simulink library "UAVdesign_net"  (Simulink 7.7)
settings: Solver=ode45  SolverMode=SingleTasking  StartTime=0.0  StopTime=10.0  RelTol=1e-3
undefined symbols (not defined in the file or in its folder): alpha_IERA_IELA_IELA, R_IERA_RA_RA
libraries: UAVdesign_net x75, simulink x13
(part 2 of 8)

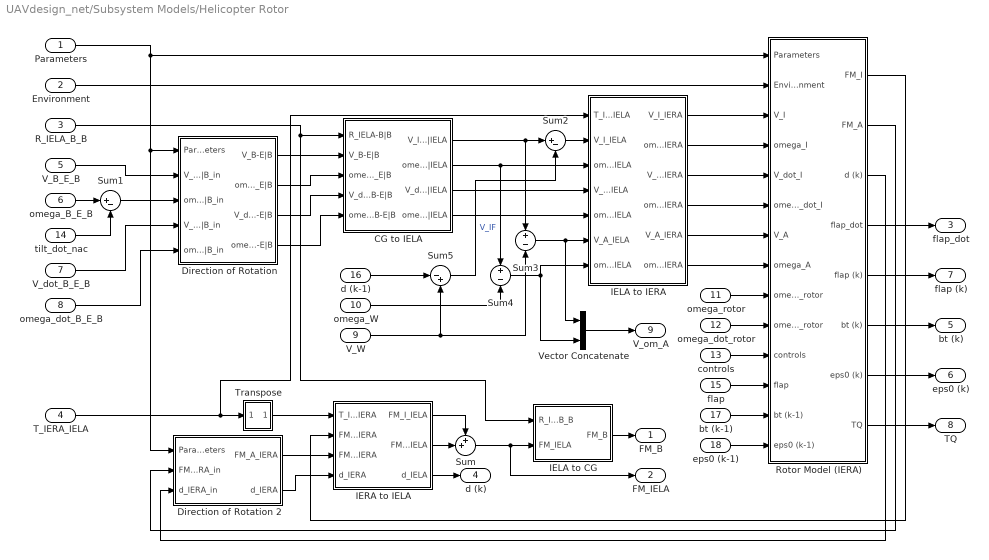
== system UAVdesign_net/Subsystem Models/Helicopter Rotor ==
  Parameters : Inport  OutDataTypeStr=Bus: RotorParameters
  Environment : Inport  Port=2  OutDataTypeStr=Bus: Environment
  R_IELA_B_B : Inport  Port=3  PortDimensions=3
  T_IERA_IELA : Inport  Port=4  PortDimensions=[3 3]
  V_B_E_B : Inport  Port=5  PortDimensions=3
  omega_B_E_B : Inport  Port=6  PortDimensions=3
  V_dot_B_E_B : Inport  Port=7  PortDimensions=3
  omega_dot_B_E_B : Inport  Port=8  PortDimensions=3
  V_W : Inport  Port=9  PortDimensions=3
  omega_W : Inport  Port=10  PortDimensions=3
  omega_rotor : Inport  Port=11  PortDimensions=1
  omega_dot_rotor : Inport  Port=12  PortDimensions=1
  controls : Inport  Port=13  PortDimensions=3
  tilt_dot_nac : Inport  Port=14  PortDimensions=3
  flap : Inport  Port=15  PortDimensions=3
  d (k-1) : Inport  Port=16  PortDimensions=3
  bt (k-1) : Inport  Port=17  PortDimensions=1
  eps0 (k-1) : Inport  Port=18  PortDimensions=1
  CG to IELA : Subsystem
      mask Display:
      | port_label('input', 1, 'R_{IELA-B|B}', 'texmode', 'on')
      | port_label('input', 2, 'V_{B-E|B}', 'texmode', 'on')
      | port_label('input', 3, '\omega_{B-E|B}', 'texmode', 'on')
      | port_label('input', 4, 'V^\bullet_{B-E|B}', 'texmode', 'on')
      | port_label('input', 5, '\omega^\bullet_{B-E|B}', 'texmode', 'on')
      | port_label('output', 1, 'V_{IELA-E|IELA}', 'texmode', 'on')
      | port_label('output', 2, '\omega_{IELA-E|IELA}', 'texmode', 'on')
      | port_label('output', 3, 'V^\bullet_{IELA-E|IELA}', 'texmode', 'on')
      | port_label('output', 4, '\omega^\bullet_{IELA-E|IELA}', 'texmode', 'on')
  Direction of Rotation : Subsystem
      mask Display:
      | port_label('input', 1, 'Parameters', 'texmode', 'on')
      | port_label('input', 2, 'V_{B-E|B}', 'texmode', 'on')
      | port_label('input', 3, '\omega_{B-E|B}', 'texmode', 'on')
      | port_label('input', 4, 'V^\bullet_{B-E|B}', 'texmode', 'on')
      | port_label('input', 5, '\omega^\bullet_{B-E|B}', 'texmode', 'on')
      | port_label('output', 1, 'V_{B-E|B}', 'texmode', 'on')
      | port_label('output', 2, '\omega_{B-E|B}', 'texmode', 'on')
      | port_label('output', 3, 'V^\bullet_{B-E|B}', 'texmode', 'on')
      | port_label('output', 4, '\omega^\bullet_{B-E|B}', 'texmode', 'on')
  Direction of Rotation 2 : Subsystem
      mask Display:
      | port_label('input', 1, 'Parameters', 'texmode', 'on')
      | port_label('input', 2, 'FM_{A|IERA}', 'texmode', 'on')
      | port_label('input', 3, 'd_{IERA}', 'texmode', 'on')
      | port_label('output', 1, 'FM_{A|IERA}', 'texmode', 'on')
      | port_label('output', 2, 'd_{IERA}', 'texmode', 'on')
  IELA to CG : Subsystem
      mask Display:
      | port_label('input', 1, 'R_{IELA-B|B}', 'texmode', 'on')
      | port_label('input', 2, 'FM_{IELA}', 'texmode', 'on')
      | port_label('output', 1, 'FM_{B}', 'texmode', 'on')
  IELA to IERA : Subsystem
      mask Display:
      | port_label('input', 1, 'T_{IERA-IELA}', 'texmode', 'on')
      | port_label('input', 2, 'V_{I|IELA}', 'texmode', 'on')
      | port_label('input', 3, '\omega_{I|IELA}', 'texmode', 'on')
      | port_label('input', 4, 'V^\bullet_{I|IELA}', 'texmode', 'on')
      | port_label('input', 5, '\omega^\bullet_{I|IELA}', 'texmode', 'on')
      | port_label('input', 6, 'V_{A|IELA}', 'texmode', 'on')
      | port_label('input', 7, '\omega_{A|IELA}', 'texmode', 'on')
      | 
      | port_label('output', 1, 'V_{I|IERA}', 'texmode', 'on')
      | port_label('output', 2, '\omega_{I|IERA}', 'texmode', 'on')
      | port_label('output', 3, 'V^\bullet_{I|IERA}', 'texmode', 'on')
      | port_label('output', 4, '\omega^\bullet_{I|IERA}', 'texmode', 'on')
      | port_label('output', 5, 'V_{A|IERA}', 'texmode', 'on')
      | port_label('output', 6, '\omega_{A|IERA}', 'texmode', 'on')
  IERA to IELA : Subsystem
      mask Display:
      | port_label('input', 1, 'T_{IELA-IERA}', 'texmode', 'on')
      | port_label('input', 2, 'FM_{I|IERA}', 'texmode', 'on')
      | port_label('input', 3, 'FM_{A|IERA}', 'texmode', 'on')
      | port_label('input', 4, 'd_{IERA}', 'texmode', 'on')
      | port_label('output', 1, 'FM_{I|IELA}', 'texmode', 'on')
      | port_label('output', 2, 'FM_{A|IELA}', 'texmode', 'on')
      | port_label('output', 3, 'd_{IELA}', 'texmode', 'on')
  Rotor Model (IERA) : Subsystem
      mask Display:
      | port_label('input', 1, 'Parameters', 'texmode', 'on')
      | port_label('input', 2, 'Environment', 'texmode', 'on')
      | port_label('input', 3, 'V_{I}', 'texmode', 'on')
      | port_label('input', 4, '\omega_{I}', 'texmode', 'on')
      | port_label('input', 5, 'V^\bullet_{I}', 'texmode', 'on')
      | port_label('input', 6, '\omega^\bullet_{I}', 'texmode', 'on')
      | port_label('input', 7, 'V_{A}', 'texmode', 'on')
      | port_label('input', 8, '\omega_{A}', 'texmode', 'on')
      | port_label('input', 9, '\Omega_{rotor}', 'texmode', 'on')
      | port_label('input', 10, '\Omega^\bullet_{rotor}', 'texmode', 'on')
      | port_label('input', 11, 'controls', 'texmode', 'on')
      | port_label('input', 12, 'flap', 'texmode', 'on')
      | port_label('input', 13, 'bt_{k-1}', 'texmode', 'on')
      | port_label('input', 14, 'eps0_{k-1}', 'texmode', 'on')
      | 
      | port_label('output', 1, 'FM_{I}', 'texmode', 'on')
      | port_label('output', 2, 'FM_{A}', 'texmode', 'on')
      | port_label('output', 3, 'd_{k}', 'texmode', 'on')
      | port_label('output', 4, 'flap^\bullet', 'texmode', 'on')
      | port_label('output', 5, 'flap_{k}', 'texmode', 'on')
      | port_label('output', 6, 'bt_{k}', 'texmode', 'on')
      | port_label('output', 7, 'eps0_{k}', 'texmode', 'on')
      | port_label('output', 8, 'Lift & Torque', 'texmode', 'on')
  Sum : Sum  Inputs=++|
  Sum1 : Sum  Inputs=|+-
  Sum2 : Sum  Inputs=|+-
  Sum3 : Sum  Inputs=+|-
  Sum4 : Sum  Inputs=+|-
  Sum5 : Sum  Inputs=|-+
  Transpose : Subsystem
      mask Display: disp('A^T', 'texmode', 'on')
  Vector Concatenate : Concatenate  Mode=Vector
  FM_B : Outport  PortDimensions=6
  FM_IELA : Outport  Port=2  PortDimensions=6
  flap_dot : Outport  Port=3  PortDimensions=3
  d (k) : Outport  Port=4  PortDimensions=3
  bt (k) : Outport  Port=5  PortDimensions=1
  eps0 (k) : Outport  Port=6  PortDimensions=1
  flap (k) : Outport  Port=7  PortDimensions=3
  TQ : Outport  Port=8  PortDimensions=2
  V_om_A : Outport  Port=9  PortDimensions=6
  wires:
  R_IELA_B_B/1 -> CG to IELA/1(R_IELA-B|B), IELA to CG/1(R_IELA_B_B)
  eps0 (k-1)/1 -> Rotor Model (IERA)/14(eps0 (k-1))
  IERA to IELA/3(d_IELA) -> d (k)/1
  Rotor Model (IERA)/7(eps0 (k)) -> eps0 (k)/1
  bt (k-1)/1 -> Rotor Model (IERA)/13(bt (k-1))
  IELA to CG/1(FM_B) -> FM_B/1
  Transpose/1(Out) -> IERA to IELA/1(T_IELA_IERA)
  Rotor Model (IERA)/6(bt (k)) -> bt (k)/1
  flap/1 -> Rotor Model (IERA)/12(flap)
  controls/1 -> Rotor Model (IERA)/11(controls)
  Rotor Model (IERA)/5(flap (k)) -> flap (k)/1
  omega_dot_rotor/1 -> Rotor Model (IERA)/10(omega_dot_rotor)
  omega_W/1 -> Sum4/2
  omega_rotor/1 -> Rotor Model (IERA)/9(omega_rotor)
  d (k-1)/1 -> Sum5/1
  Rotor Model (IERA)/4(flap_dot) -> flap_dot/1
  omega_dot_B_E_B/1 -> Direction of Rotation/5(omega_dot_B-E|B_in)
  tilt_dot_nac/1 -> Sum1/2
  V_dot_B_E_B/1 -> Direction of Rotation/4(V_dot_B-E|B_in)
  omega_B_E_B/1 -> Sum1/1
  V_B_E_B/1 -> Direction of Rotation/2(V_B-E|B_in)
  T_IERA_IELA/1 -> Transpose/1(In), IELA to IERA/1(T_IERA_IELA)
  Environment/1 -> Rotor Model (IERA)/2(Environment)
  Parameters/1 -> Direction of Rotation 2/1(Parameters), Direction of Rotation/1(Parameters), Rotor Model (IERA)/1(Parameters)
  Direction of Rotation 2/2(d_IERA) -> IERA to IELA/4(d_IERA)
  Rotor Model (IERA)/3(d (k)) -> Direction of Rotation 2/3(d_IERA_in)
  Sum5/1 -> Sum2/2  "V_IF"
  Direction of Rotation 2/1(FM_A_IERA) -> IERA to IELA/3(FM_A_IERA)
  IERA to IELA/2(FM_A_IELA) -> Sum/2
  IELA to IERA/6(omega_A_IERA) -> Rotor Model (IERA)/8(omega_A)
  IELA to IERA/5(V_A_IERA) -> Rotor Model (IERA)/7(V_A)
  IELA to IERA/4(omega_dot_I_IERA) -> Rotor Model (IERA)/6(omega_dot_I)
  IELA to IERA/3(V_dot_I_IERA) -> Rotor Model (IERA)/5(V_dot_I)
  IELA to IERA/2(omega_I_IERA) -> Rotor Model (IERA)/4(omega_I)
  IELA to IERA/1(V_I_IERA) -> Rotor Model (IERA)/3(V_I)
  Sum4/1 -> IELA to IERA/7(omega_A_IELA), Vector Concatenate/2
  V_W/1 -> Sum5/2, Sum3/2
  Sum3/1 -> IELA to IERA/6(V_A_IELA), Vector Concatenate/1
  Sum2/1 -> IELA to IERA/2(V_I_IELA)
  CG to IELA/1(V_IELA-E|IELA) -> Sum3/1, Sum2/1
  Direction of Rotation/4(omega_dot_B-E|B) -> CG to IELA/5(omega_dot_B-E|B)
  Direction of Rotation/3(V_dot_B-E|B) -> CG to IELA/4(V_dot_B-E|B)
  Direction of Rotation/2(omega_B_E|B) -> CG to IELA/3(omega_B_E|B)
  Direction of Rotation/1(V_B-E|B) -> CG to IELA/2(V_B-E|B)
  Sum1/1 -> Direction of Rotation/3(omega_B_E|B_in)
  Rotor Model (IERA)/1(FM_I) -> IERA to IELA/2(FM_I_IERA)
  Rotor Model (IERA)/2(FM_A) -> Direction of Rotation 2/2(FM_A_IERA_in)
  Sum/1 -> IELA to CG/2(FM_IELA), FM_IELA/1
  IERA to IELA/1(FM_I_IELA) -> Sum/1
  CG to IELA/4(omega_dot_IELA-E|IELA) -> IELA to IERA/5(omega_dot_I_IELA)
  CG to IELA/3(V_dot_IELA-E|IELA) -> IELA to IERA/4(V_dot_I_IELA)
  CG to IELA/2(omega_IELA-E|IELA) -> Sum4/1, IELA to IERA/3(omega_I_IELA)
  Rotor Model (IERA)/8(TQ) -> TQ/1
  Vector Concatenate/1 -> V_om_A/1

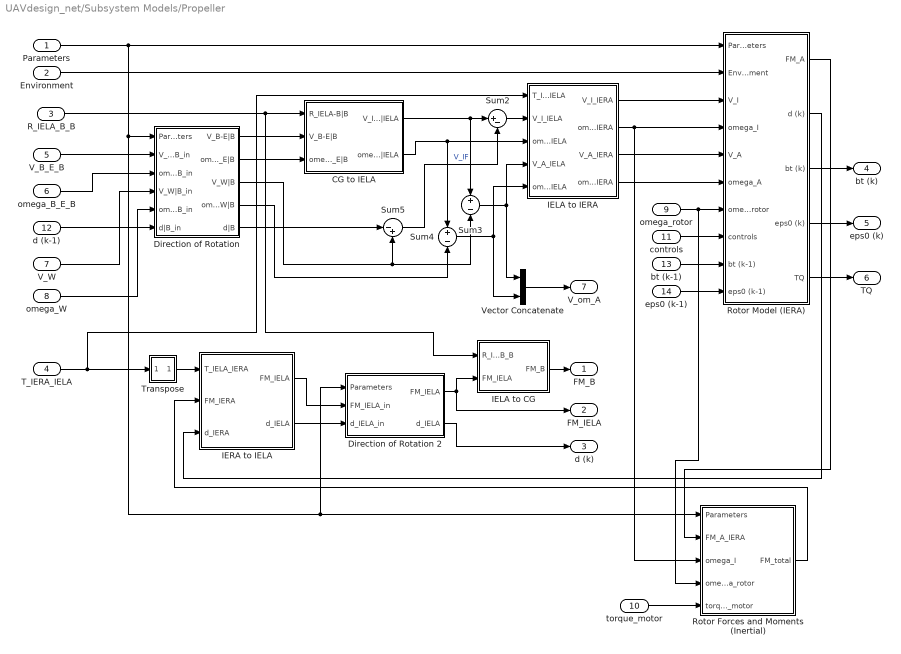
== system UAVdesign_net/Subsystem Models/Propeller ==
  Parameters : Inport
  Environment : Inport  Port=2
  R_IELA_B_B : Inport  Port=3  PortDimensions=3
  T_IERA_IELA : Inport  Port=4  PortDimensions=[3 3]
  V_B_E_B : Inport  Port=5  PortDimensions=3
  omega_B_E_B : Inport  Port=6  PortDimensions=3
  V_W : Inport  Port=7  PortDimensions=3
  omega_W : Inport  Port=8  PortDimensions=3
  omega_rotor : Inport  Port=9  PortDimensions=1
  torque_motor : Inport  Port=10  PortDimensions=1
  controls : Inport  Port=11  PortDimensions=1
  d (k-1) : Inport  Port=12  PortDimensions=3
  bt (k-1) : Inport  Port=13  PortDimensions=1
  eps0 (k-1) : Inport  Port=14  PortDimensions=1
  CG to IELA : Subsystem
      mask Display:
      | port_label('input', 1, 'R_{IELA-B|B}', 'texmode', 'on')
      | port_label('input', 2, 'V_{B-E|B}', 'texmode', 'on')
      | port_label('input', 3, '\omega_{B-E|B}', 'texmode', 'on')
      | port_label('output', 1, 'V_{IELA-E|IELA}', 'texmode', 'on')
      | port_label('output', 2, '\omega_{IELA-E|IELA}', 'texmode', 'on')
  Direction of Rotation : Subsystem
      mask Display:
      | port_label('input', 1, 'Parameters', 'texmode', 'on')
      | port_label('input', 2, 'V_{B-E|B}', 'texmode', 'on')
      | port_label('input', 3, '\omega_{B-E|B}', 'texmode', 'on')
      | port_label('input', 4, 'V_{W|B}', 'texmode', 'on')
      | port_label('input', 5, '\omega_{W|B}', 'texmode', 'on')
      | port_label('input', 6, 'd', 'texmode', 'on')
      | 
      | port_label('output', 1, 'V_{B-E|B}', 'texmode', 'on')
      | port_label('output', 2, '\omega_{B-E|B}', 'texmode', 'on')
      | port_label('output', 3, 'V_{W|B}', 'texmode', 'on')
      | port_label('output', 4, '\omega_{W|B}', 'texmode', 'on')
      | port_label('output', 5, 'd', 'texmode', 'on')
  Direction of Rotation 2 : Subsystem
      mask Display:
      | port_label('input', 1, 'Parameters', 'texmode', 'on')
      | port_label('input', 2, 'FM_{IELA}', 'texmode', 'on')
      | port_label('input', 3, 'd_{IELA}', 'texmode', 'on')
      | port_label('output', 1, 'FM_{IELA}', 'texmode', 'on')
      | port_label('output', 2, 'd_{IELA}', 'texmode', 'on')
  IELA to CG : Subsystem
      mask Display:
      | port_label('input', 1, 'R_{IELA-B|B}', 'texmode', 'on')
      | port_label('input', 2, 'FM_{IELA}', 'texmode', 'on')
      | port_label('output', 1, 'FM_{B}', 'texmode', 'on')
  IELA to IERA : Subsystem
      mask Display:
      | port_label('input', 1, 'T_{IERA-IELA}', 'texmode', 'on')
      | port_label('input', 2, 'V_{I|IELA}', 'texmode', 'on')
      | port_label('input', 3, '\omega_{I|IELA}', 'texmode', 'on')
      | port_label('input', 4, 'V_{A|IELA}', 'texmode', 'on')
      | port_label('input', 5, '\omega_{A|IELA}', 'texmode', 'on')
      | 
      | port_label('output', 1, 'V_{I|IERA}', 'texmode', 'on')
      | port_label('output', 2, '\omega_{I|IERA}', 'texmode', 'on')
      | port_label('output', 3, 'V_{A|IERA}', 'texmode', 'on')
      | port_label('output', 4, '\omega_{A|IERA}', 'texmode', 'on')
  IERA to IELA : Subsystem
      mask Display:
      | port_label('input', 1, 'T_{IELA-IERA}', 'texmode', 'on')
      | port_label('input', 2, 'FM_{IERA}', 'texmode', 'on')
      | port_label('input', 3, 'd_{IERA}', 'texmode', 'on')
      | port_label('output', 1, 'FM_{IELA}', 'texmode', 'on')
      | port_label('output', 2, 'd_{IELA}', 'texmode', 'on')
  Rotor Forces and Moments (Inertial) : Subsystem
      mask Display:
      | port_label('input', 1, 'Parameters', 'texmode', 'on')
      | port_label('input', 2, 'FM_{A|IERA}', 'texmode', 'on')
      | port_label('input', 3, '\omega_{I|IERA}', 'texmode', 'on')
      | port_label('input', 4, '\Omega_{rotor}', 'texmode', 'on')
      | port_label('input', 5, '\tau_{motor}', 'texmode', 'on')
      | 
      | port_label('output', 1, 'FM_{total|IERA}', 'texmode', 'on')
  Rotor Model (IERA) : Subsystem
      mask Display:
      | port_label('input', 1, 'Parameters', 'texmode', 'on')
      | port_label('input', 2, 'Environment', 'texmode', 'on')
      | port_label('input', 3, 'V_{I}', 'texmode', 'on')
      | port_label('input', 4, '\omega_{I}', 'texmode', 'on')
      | port_label('input', 5, 'V_{A}', 'texmode', 'on')
      | port_label('input', 6, '\omega_{A}', 'texmode', 'on')
      | port_label('input', 7, '\Omega_{rotor}', 'texmode', 'on')
      | port_label('input', 8, 'controls', 'texmode', 'on')
      | port_label('input', 9, 'bt_{k-1}', 'texmode', 'on')
      | port_label('input', 10, 'eps0_{k-1}', 'texmode', 'on')
      | 
      | port_label('output', 1, 'FM_{A}', 'texmode', 'on')
      | port_label('output', 2, 'd_{k}', 'texmode', 'on')
      | port_label('output', 3, 'bt_{k}', 'texmode', 'on')
      | port_label('output', 4, 'eps0_{k}', 'texmode', 'on')
      | port_label('output', 5, 'Lift & Torque', 'texmode', 'on')
  Sum2 : Sum  Inputs=|+-
  Sum3 : Sum  Inputs=+|-
  Sum4 : Sum  Inputs=+|-
  Sum5 : Sum  Inputs=|-+
  Transpose : Subsystem
      mask Display: disp('A^T', 'texmode', 'on')
  Vector Concatenate : Concatenate  Mode=Vector
  FM_B : Outport  PortDimensions=6
  FM_IELA : Outport  Port=2  PortDimensions=6
  d (k) : Outport  Port=3  PortDimensions=3
  bt (k) : Outport  Port=4  PortDimensions=1
  eps0 (k) : Outport  Port=5  PortDimensions=1
  TQ : Outport  Port=6  PortDimensions=2
  V_om_A : Outport  Port=7  PortDimensions=6
  wires:
  Vector Concatenate/1 -> V_om_A/1
  Rotor Model (IERA)/5(TQ) -> TQ/1
  CG to IELA/2(omega_IELA-E|IELA) -> IELA to IERA/3(omega_I_IELA), Sum4/1
  Rotor Model (IERA)/1(FM_A) -> Rotor Forces and Moments (Inertial)/2(FM_A_IERA)
  Direction of Rotation/1(V_B-E|B) -> CG to IELA/2(V_B-E|B)
  Direction of Rotation/2(omega_B_E|B) -> CG to IELA/3(omega_B_E|B)
  CG to IELA/1(V_IELA-E|IELA) -> Sum2/1, Sum3/1
  Sum2/1 -> IELA to IERA/2(V_I_IELA)
  Sum3/1 -> Vector Concatenate/1, IELA to IERA/4(V_A_IELA)
  Sum4/1 -> Vector Concatenate/2, IELA to IERA/5(omega_A_IELA)
  IELA to IERA/1(V_I_IERA) -> Rotor Model (IERA)/3(V_I)
  IELA to IERA/2(omega_I_IERA) -> Rotor Model (IERA)/4(omega_I), Rotor Forces and Moments (Inertial)/3(omega_I)
  IELA to IERA/3(V_A_IERA) -> Rotor Model (IERA)/5(V_A)
  IELA to IERA/4(omega_A_IERA) -> Rotor Model (IERA)/6(omega_A)
  Sum5/1 -> Sum2/2  "V_IF"
  Rotor Model (IERA)/2(d (k)) -> IERA to IELA/3(d_IERA)
  Parameters/1 -> Rotor Model (IERA)/1(Parameters), Direction of Rotation/1(Parameters), Rotor Forces and Moments (Inertial)/1(Parameters), Direction of Rotation 2/1(Parameters)
  Environment/1 -> Rotor Model (IERA)/2(Environment)
  T_IERA_IELA/1 -> IELA to IERA/1(T_IERA_IELA), Transpose/1(In)
  V_B_E_B/1 -> Direction of Rotation/2(V_B-E|B_in)
  omega_B_E_B/1 -> Direction of Rotation/3(omega_B_E|B_in)
  omega_rotor/1 -> Rotor Model (IERA)/7(omega_rotor), Rotor Forces and Moments (Inertial)/4(omega_rotor)
  controls/1 -> Rotor Model (IERA)/8(controls)
  Rotor Model (IERA)/3(bt (k)) -> bt (k)/1
  Transpose/1(Out) -> IERA to IELA/1(T_IELA_IERA)
  IELA to CG/1(FM_B) -> FM_B/1
  bt (k-1)/1 -> Rotor Model (IERA)/9(bt (k-1))
  Rotor Model (IERA)/4(eps0 (k)) -> eps0 (k)/1
  eps0 (k-1)/1 -> Rotor Model (IERA)/10(eps0 (k-1))
  R_IELA_B_B/1 -> IELA to CG/1(R_IELA_B_B), CG to IELA/1(R_IELA-B|B)
  torque_motor/1 -> Rotor Forces and Moments (Inertial)/5(torque_motor)
  Rotor Forces and Moments (Inertial)/1(FM_total) -> IERA to IELA/2(FM_IERA)
  IERA to IELA/2(d_IELA) -> Direction of Rotation 2/3(d_IELA_in)
  IERA to IELA/1(FM_IELA) -> Direction of Rotation 2/2(FM_IELA_in)
  Direction of Rotation 2/1(FM_IELA) -> IELA to CG/2(FM_IELA), FM_IELA/1
  Direction of Rotation 2/2(d_IELA) -> d (k)/1
  d (k-1)/1 -> Direction of Rotation/6(d|B_in)
  Direction of Rotation/5(d|B) -> Sum5/1
  omega_W/1 -> Direction of Rotation/5(omega_W|B_in)
  Direction of Rotation/4(omega_W|B) -> Sum4/2
  V_W/1 -> Direction of Rotation/4(V_W|B_in)
  Direction of Rotation/3(V_W|B) -> Sum3/2, Sum5/2

== system UAVdesign_net/Subsystem Models/Propeller Rotation Dynamics ==
  Parameters : Inport
  T_IERA_IELA : Inport  Port=2  PortDimensions=[3 3]
  torque_prop : Inport  Port=3
  torque_motor : Inport  Port=4
  omega_I : Inport  Port=5
  omega_dot_I : Inport  Port=6
  omega_rotor : Inport  Port=7
  Direction of Rotation : Subsystem
      mask Display:
      | port_label('input', 1, 'Parameters', 'texmode', 'on')
      | port_label('input', 2, '\omega_{B-E|B}', 'texmode', 'on')
      | port_label('input', 3, '\omega^\bullet_{B-E|B}', 'texmode', 'on')
      | port_label('output', 1, '\omega_{B-E|B}', 'texmode', 'on')
      | port_label('output', 2, '\omega^\bullet_{B-E|B}', 'texmode', 'on')
  IELA to IERA : Subsystem
      mask Display:
      | port_label('input', 1, 'T_{IERA-IELA}', 'texmode', 'on')
      | port_label('input', 2, '\omega_{I|IELA}', 'texmode', 'on')
      | port_label('input', 3, '\omega^\bullet_{I|IELA}', 'texmode', 'on')
      | 
      | port_label('output', 1, '\omega_{I|IERA}', 'texmode', 'on')
      | port_label('output', 2, '\omega^\bullet_{I|IERA}', 'texmode', 'on')
  Propeller rotation dynamics : Stateflow chart  TreatAsAtomicUnit=on
  omega_dot_rotor : Outport  PortDimensions=1
  wires:
  omega_dot_I/1 -> Direction of Rotation/3(omega_dot_B_E|B_in)
  Propeller rotation dynamics/1(omegad) -> omega_dot_rotor/1
  torque_motor/1 -> Propeller rotation dynamics/5(tau_motor)
  omega_rotor/1 -> Propeller rotation dynamics/4(omega)
  Parameters/1 -> Propeller rotation dynamics/1(Parameters), Direction of Rotation/1(Parameters)
  omega_I/1 -> Direction of Rotation/2(omega_B_E|B_in)
  torque_prop/1 -> Propeller rotation dynamics/6(tau_prop)
  Direction of Rotation/1(omega_B_E|B) -> IELA to IERA/2(omega_I_IELA)
  Direction of Rotation/2(omega_dot_B_E|B) -> IELA to IERA/3(omega_dot_I_IELA)
  T_IERA_IELA/1 -> IELA to IERA/1(T_IERA_IELA)
  IELA to IERA/1(omega_I_IERA) -> Propeller rotation dynamics/2(omi)
  IELA to IERA/2(omega_dot_I_IERA) -> Propeller rotation dynamics/3(omid)

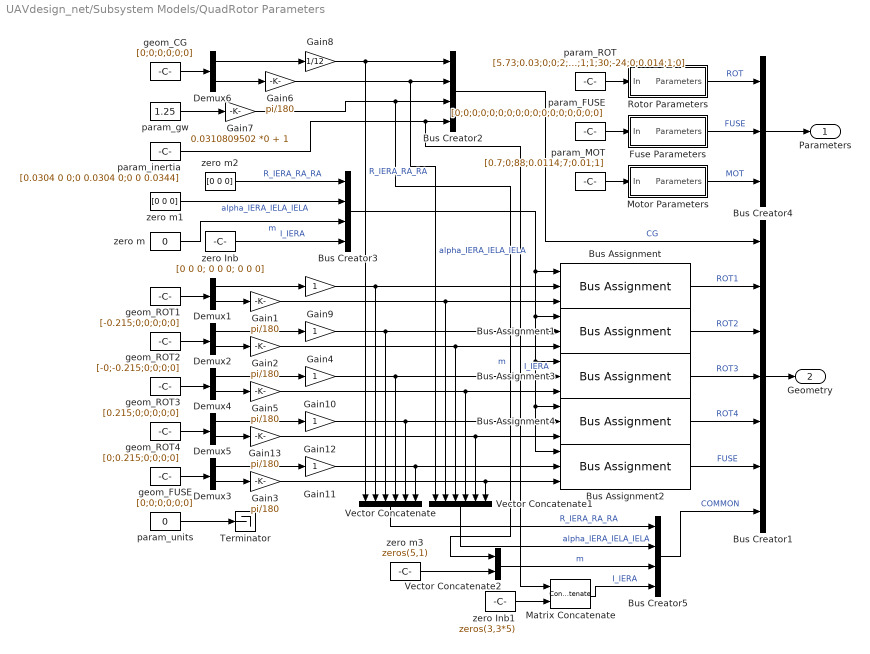
== system UAVdesign_net/Subsystem Models/QuadRotor Parameters ==
  Bus Assignment{,1..4} (5 alike) : BusAssignment  AssignedSignals=R_IERA_RA_RA,alpha_IERA_IELA_IELA
  Bus Creator1 : BusCreator  Inputs=7
  Bus Creator2 : BusCreator
  Bus Creator3 : BusCreator
  Bus Creator4 : BusCreator  Inputs=3
  Bus Creator5 : BusCreator
  Demux{1..6} (6 alike) : Demux  Outputs=2
  Fuse Parameters : Subsystem
  Gain{1..3,5..6,13} (6 alike) : Gain  Gain=pi/180
  Gain{4,9..12} (5 alike) : Gain
  Gain7 : Gain  Gain=0.0310809502 *0 + 1
  Gain8 : Gain  Gain=1/12
  Matrix Concatenate : Concatenate  Mode=Multidimensional array  ConcatenateDimension=2
  Motor Parameters : Subsystem
  Rotor Parameters : Subsystem
  Terminator : Terminator
  Vector Concatenate : Concatenate  NumInputs=6  Mode=Vector
  Vector Concatenate1 : Concatenate  NumInputs=6  Mode=Vector
  Vector Concatenate2 : Concatenate  Mode=Vector
  geom_CG : Constant  Value=[0;0;0;0;0;0]
  geom_FUSE : Constant  Value=[0;0;0;0;0;0]
  geom_ROT1 : Constant  Value=[-0.215;0;0;0;0;0]
  geom_ROT2 : Constant  Value=[-0;-0.215;0;0;0;0]
  geom_ROT3 : Constant  Value=[0.215;0;0;0;0;0]
  geom_ROT4 : Constant  Value=[0;0.215;0;0;0;0]
  param_FUSE : Constant  Value=[0;0;0;0;0;0;0;0;0;0;0;0;0;0;0;0;0]
  param_MOT : Constant  Value=[0.7;0;88;0.0114;7;0.01;1]
  param_ROT : Constant  Value=[5.73;0.03;0;0;2;0.127;0.016;0.95;1;1;30;-24;0;0.014;1;0]
  param_gw : Constant  Value=1.25
  param_inertia : Constant  Value=[0.0304 0 0;0 0.0304 0;0 0 0.0344]
  param_units : Constant  Value=0
  zero Inb : Constant  Value=[0 0 0; 0 0 0; 0 0 0]
  zero Inb1 : Constant  Value=zeros(3,3*5)
  zero m : Constant  Value=0
  zero m1 : Constant  Value=[0 0 0]
  zero m2 : Constant  Value=[0 0 0]
  zero m3 : Constant  Value=zeros(5,1)
  Parameters : Outport
  Geometry : Outport  Port=2
  wires:
  zero m3/1 -> Vector Concatenate2/2
  Vector Concatenate2/1 -> Bus Creator5/3  "m"
  Bus Creator1/1 -> Geometry/1
  Demux6/1 -> Gain8/1
  Demux6/2 -> Gain6/1
  param_gw/1 -> Gain7/1
  Demux1/1 -> Gain9/1
  Demux1/2 -> Gain1/1
  geom_ROT1/1 -> Demux1/1
  Demux3/1 -> Gain11/1
  Demux3/2 -> Gain3/1
  geom_FUSE/1 -> Demux3/1
  geom_CG/1 -> Demux6/1
  Bus Creator3/1 -> Bus Assignment/1, Bus Assignment1/1, Bus Assignment3/1, Bus Assignment2/1, Bus Assignment4/1
  Bus Creator4/1 -> Parameters/1
  param_ROT/1 -> Rotor Parameters/1(In)
  param_FUSE/1 -> Fuse Parameters/1(In)
  Gain1/1 -> Bus Assignment/3, Vector Concatenate1/2
  Gain3/1 -> Bus Assignment2/3, Vector Concatenate1/6
  Gain11/1 -> Bus Assignment2/2, Vector Concatenate/6
  Bus Assignment2/1 -> Bus Creator1/6  "FUSE"
  Bus Assignment/1 -> Bus Creator1/2  "ROT1"
  Bus Creator2/1 -> Bus Creator1/1  "CG"
  zero m2/1 -> Bus Creator3/1  "R_IERA_RA_RA"
  zero m1/1 -> Bus Creator3/2  "alpha_IERA_IELA_IELA"
  param_units/1 -> Terminator/1
  Rotor Parameters/1(Parameters) -> Bus Creator4/1  "ROT"
  Fuse Parameters/1(Parameters) -> Bus Creator4/2  "FUSE"
  Gain8/1 -> Bus Creator2/1, Vector Concatenate/1  "R_IERA_RA_RA"
  Gain6/1 -> Bus Creator2/2, Vector Concatenate1/1  "alpha_IERA_IELA_IELA"
  zero Inb/1 -> Bus Creator3/4  "I_IERA"
  zero m/1 -> Bus Creator3/3  "m"
  Gain7/1 -> Vector Concatenate2/1, Bus Creator2/3  "m"
  param_inertia/1 -> Bus Creator2/4, Matrix Concatenate/1  "I_IERA"
  Demux2/1 -> Gain4/1
  Demux2/2 -> Gain2/1
  Gain2/1 -> Bus Assignment1/3, Vector Concatenate1/3
  Gain4/1 -> Bus Assignment1/2, Vector Concatenate/3
  geom_ROT2/1 -> Demux2/1
  Gain9/1 -> Bus Assignment/2, Vector Concatenate/2
  Demux4/1 -> Gain10/1
  Demux4/2 -> Gain5/1
  Gain5/1 -> Bus Assignment3/3, Vector Concatenate1/4
  Gain10/1 -> Bus Assignment3/2, Vector Concatenate/4
  geom_ROT3/1 -> Demux4/1
  Demux5/1 -> Gain12/1
  Demux5/2 -> Gain13/1
  Gain13/1 -> Bus Assignment4/3, Vector Concatenate1/5
  Gain12/1 -> Bus Assignment4/2, Vector Concatenate/5
  geom_ROT4/1 -> Demux5/1
  Bus Assignment1/1 -> Bus Creator1/3  "ROT2"
  Bus Assignment3/1 -> Bus Creator1/4  "ROT3"
  Bus Assignment4/1 -> Bus Creator1/5  "ROT4"
  Bus Creator5/1 -> Bus Creator1/7  "COMMON"
  Vector Concatenate1/1 -> Bus Creator5/2  "alpha_IERA_IELA_IELA"
  Matrix Concatenate/1 -> Bus Creator5/4  "I_IERA"
  Vector Concatenate/1 -> Bus Creator5/1  "R_IERA_RA_RA"
  zero Inb1/1 -> Matrix Concatenate/2
  param_MOT/1 -> Motor Parameters/1(In)
  Motor Parameters/1(Parameters) -> Bus Creator4/3  "MOT"

== system UAVdesign_net/Subsystem Models/Wing ==
  Parameters : Inport  OutDataTypeStr=Bus: FinParameters
  Environment : Inport  Port=2  OutDataTypeStr=Bus: Environment
  R_IELA_B_B : Inport  Port=3  PortDimensions=3
  T_IERA_IELA : Inport  Port=4  PortDimensions=[3 3]
  V_B_E_B : Inport  Port=5  PortDimensions=3
  omega_B_E_B : Inport  Port=6  PortDimensions=3
  V_W : Inport  Port=7  PortDimensions=3
  omega_W : Inport  Port=8  PortDimensions=3
  CG to IELA : Subsystem
      mask Display:
      | port_label('input', 1, 'R_{IELA-B|B}', 'texmode', 'on')
      | port_label('input', 2, 'V_{B-E|B}', 'texmode', 'on')
      | port_label('input', 3, '\omega_{B-E|B}', 'texmode', 'on')
      | port_label('output', 1, 'V_{IELA-E|IELA}', 'texmode', 'on')
      | port_label('output', 2, '\omega_{IELA-E|IELA}', 'texmode', 'on')
  IELA to CG : Subsystem
      mask Display:
      | port_label('input', 1, 'R_{IELA-B|B}', 'texmode', 'on')
      | port_label('input', 2, 'FM_{IELA}', 'texmode', 'on')
      | port_label('output', 1, 'FM_{B}', 'texmode', 'on')
  IELA to IERA : Subsystem
      mask Display:
      | port_label('input', 1, 'T_{IERA-IELA}', 'texmode', 'on')
      | port_label('input', 2, 'V_{A|IELA}', 'texmode', 'on')
      | port_label('input', 3, '\omega_{A|IELA}', 'texmode', 'on')
      | port_label('input', 4, 'V_{W|IELA}', 'texmode', 'on')
      | port_label('input', 5, '\omega_{W|IELA}', 'texmode', 'on')
      | 
      | port_label('output', 1, 'V_{A|IERA}', 'texmode', 'on')
      | port_label('output', 2, '\omega_{A|IERA}', 'texmode', 'on')
      | port_label('output', 3, 'V_{W|IERA}', 'texmode', 'on')
      | port_label('output', 4, '\omega_{W|IERA}', 'texmode', 'on')
  IERA to IELA : Subsystem
      mask Display:
      | port_label('input', 1, 'T_{IELA-IERA}', 'texmode', 'on')
      | port_label('input', 2, 'FM_{I|IERA}', 'texmode', 'on')
      | port_label('input', 3, 'FM_{A|IERA}', 'texmode', 'on')
      | port_label('input', 4, 'd_{IERA}', 'texmode', 'on')
      | port_label('output', 1, 'FM_{I|IELA}', 'texmode', 'on')
      | port_label('output', 2, 'FM_{A|IELA}', 'texmode', 'on')
      | port_label('output', 3, 'd_{IELA}', 'texmode', 'on')
  No control : Constant  Value=0
  Sum : Sum  Inputs=++|
  Sum3 : Sum  Inputs=|+-
  Sum4 : Sum  Inputs=|+-
  Transpose : Subsystem
      mask Display: disp('A^T', 'texmode', 'on')
  Vector Concatenate : Concatenate  Mode=Vector
  Wing Model (IERA) : Subsystem
      mask Display:
      | port_label('input', 1, 'Parameters', 'texmode', 'on')
      | port_label('input', 2, 'Environment', 'texmode', 'on')
      | port_label('input', 3, 'V_{A}', 'texmode', 'on')
      | port_label('input', 4, '\omega_{A}', 'texmode', 'on')
      | port_label('input', 5, 'V_{W}', 'texmode', 'on')
      | port_label('input', 6, '\omega_{W}', 'texmode', 'on')
      | port_label('input', 7, 'control', 'texmode', 'on')
      | 
      | port_label('output', 1, 'FM_{I}', 'texmode', 'on')
      | port_label('output', 2, 'FM_{A}', 'texmode', 'on')
      | port_label('output', 3, 'd_{k}', 'texmode', 'on')
  FM_B : Outport  PortDimensions=6
  FM_IELA : Outport  Port=2  PortDimensions=6
  d (k) : Outport  Port=3  PortDimensions=3
  V_om_A : Outport  Port=4  PortDimensions=6
  wires:
  No control/1 -> Wing Model (IERA)/7(control)
  omega_W/1 -> IELA to IERA/5(omega_W_IELA), Sum4/2
  V_W/1 -> IELA to IERA/4(V_W_IELA), Sum3/2
  Sum4/1 -> IELA to IERA/3(omega_A_IELA), Vector Concatenate/2
  CG to IELA/2(omega_IELA-E|IELA) -> Sum4/1
  Sum3/1 -> IELA to IERA/2(V_A_IELA), Vector Concatenate/1
  CG to IELA/1(V_IELA-E|IELA) -> Sum3/1
  R_IELA_B_B/1 -> IELA to CG/1(R_IELA_B_B), CG to IELA/1(R_IELA-B|B)
  IERA to IELA/3(d_IELA) -> d (k)/1
  IELA to CG/1(FM_B) -> FM_B/1
  Transpose/1(Out) -> IERA to IELA/1(T_IELA_IERA)
  V_B_E_B/1 -> CG to IELA/2(V_B-E|B)
  T_IERA_IELA/1 -> Transpose/1(In), IELA to IERA/1(T_IERA_IELA)
  Environment/1 -> Wing Model (IERA)/2(Environment)
  Parameters/1 -> Wing Model (IERA)/1(Parameters)
  Wing Model (IERA)/3(d (k)) -> IERA to IELA/4(d_IERA)
  IERA to IELA/2(FM_A_IELA) -> Sum/2
  IELA to IERA/4(omega_W_IERA) -> Wing Model (IERA)/6(omega_W)
  IELA to IERA/3(V_W_IERA) -> Wing Model (IERA)/5(V_W)
  IELA to IERA/2(omega_A_IERA) -> Wing Model (IERA)/4(omega_A)
  IELA to IERA/1(V_A_IERA) -> Wing Model (IERA)/3(V_A)
  omega_B_E_B/1 -> CG to IELA/3(omega_B_E|B)
  Wing Model (IERA)/1(FM_I) -> IERA to IELA/2(FM_I_IERA)
  Wing Model (IERA)/2(FM_A) -> IERA to IELA/3(FM_A_IERA)
  Sum/1 -> IELA to CG/2(FM_IELA), FM_IELA/1
  IERA to IELA/1(FM_I_IELA) -> Sum/1
  Vector Concatenate/1 -> V_om_A/1

== system UAVdesign_net/Utilities/Axes ==
  Attitude Estimation : Subsystem
      mask Type: Attitude Estimation
      mask Description:
      | ESOQ2 Attitude Estimation algorithm.
      | 
      | It uses the known values of two vectors resolved to Earth axes (NED) and the measured values for the same two vectors resolved to body axes.
      | 
      | Ve1, Vb1 and a1 are the Earth value, Body value and weight for the first vector.
      | 
      | Ve2, Vb2 and a2 are the Earth value, Body value and weight for the second vector.
      mask Display:
      | port_label('input',1,'V_e1','texmode','on');
      | port_label('input',2,'V_b1','texmode','on');
      | port_label('input',3,'a1','texmode','on');
      | port_label('input',4,'V_e2','texmode','on');
      | port_label('input',5,'V_b2','texmode','on');
      | port_label('input',6,'a2','texmode','on');
      | port_label('output',1,'q_{opt}','texmode','on');
  Euler Rotation Matrix from Body to Earth : Subsystem
      mask Type: Ang2EulerRotMatrix
      mask Description:
      | Determine the 3-by-3 inverse Euler rotation matrix from a given set of Euler rotation angles.
      | Rotation Matrix from Body to Earth
      mask Display:
      | port_label('input',1,'[\phi,\theta,\psi]','texmode','on')
      | port_label('output',1,'T_{EB}(3x3)','texmode','on')
  Euler Rotation Matrix from Earth to Body : Subsystem
      mask Type: Ang2EulerRotMatrix
      mask Description:
      | Determine the 3-by-3 Euler rotation matrix from a given set of Euler rotation angles.
      | Rotation Matrix from Earth to Body.
      mask Display:
      | port_label('input',1,'[\phi,\theta,\psi]','texmode','on')
      | port_label('output',1,'T_{BE}(3x3)','texmode','on')
  Quaternions to Rotation Angles : Subsystem
      mask Type: QuaternionToAngle
      mask Description: Determine rotation vector from quaternion.
      mask Display:
      | port_label('input',1,'q','texmode','on')
      | port_label('output',1,'[\phi,\theta,\psi]','texmode','on')
  Rotation Angles to Quaternions : Subsystem
      mask Type: AngleToQuaternion
      mask Description: Calculate quaternion from rotation angles.
      mask Display:
      | port_label('input',1,'[\phi,\theta,\psi]','texmode','on')
      | port_label('output',1,'q','texmode','on')
  Rotation Matrix for angular rates Body to Earth : Subsystem
      mask Type: Ang2EulerRotMatrix
      mask Description:
      | Determine the 3-by-3 Euler rotation matrix for angular rates from a given set of Euler rotation angles for angular rates.
      | Rotation Matrix for angular rates from Body to Earth
      mask Display:
      | port_label('input',1,'[\phi,\theta,\psi]','texmode','on')
      | port_label('output',1,'E_{EB}(3x3)','texmode','on')
  Rotation Matrix for angular rates from Earth to Body : Subsystem
      mask Type: Ang2EulerRotMatrix
      mask Description:
      | Determine the 3-by-3 Euler rotation matrix for angular rates from a given set of Euler rotation angles for angular rates.
      | Rotation Matrix for angular rates from Earth to Body
      mask Display:
      | port_label('input',1,'[\phi,\theta,\psi]','texmode','on')
      | port_label('output',1,'E_{BE}(3x3)','texmode','on')

== system UAVdesign_net/Utilities/Continuous ==
  CD Integrator : S-Function  FunctionName=cd_integrator  Parameters=algorithm, param_source, initial_time, final_time, reset_type, x0_source, x0, output_time, limit_output, upper_sat, lower_sat, q_index, omega_dot_index, sample_time  EnableBusSupport=off  mask(CD_Integrator){algorithm=Euler, param_source=Discrete steps of the model, initial_time=0, final_time=10, reset_type=None, x0_source=Internal, x0=0, output_time=off, limit_output=off, upper_sat=inf, lower_sat=-inf, q_index=[], omega_dot_index=[], sample_time=-1}
      mask prompts: algorithm "Integration Algorithm"; param_source "Integration limits"; initial_time "Initial time"; final_time "Final time"; reset_type "Reset signal"; x0_source "Source for the initial conditions"; x0 "Initial conditions"; output_time "Have time as an output"; limit_output "Limit output"; upper_sat "Upper saturation limit"; lower_sat "Lower saturation limit"; q_index "Quaternion index interval"; omega_dot_index "Omega dot index interval"; sample_time "Sample time"
      mask help:
      | Integrator block that uses a function-call mechanism to do integration.
      | It can integrate for one simulation step or it can integrate independently of Simulink for a specified interval.
      | If no quaternion is integrated, set the quaternion interval to [].
      | If omega_dot is not used to improve the quaternion integration, set its interval limits to [].
      mask init:
      | cd_integrator_callback(gcb, 10);
      mask StyleString: popup(Euler|Runge-Kutta),popup(Discrete steps of the model|Internal|External),edit,edit,popup(None|External),popup(Internal|External),edit,checkbox,checkbox,edit,edit,edit,edit,edit
      mask CallbackString: |cd_integrator_callback(gcb, 1)||||cd_integrator_callback(gcb, 2)|||cd_integrator_callback(gcb, 3)|||||
      mask Display: disp('\fontsize{16}\int', 'texmode', 'on'); port_label('input', 1, 'x^{\bullet}', 'texmode', 'on'); port_label('output', 1, 'fn', 'texmode', 'on'); port_label('output', 2, 'x');
  Remote Execution Code : Stateflow chart  TreatAsAtomicUnit=on
      settings: CopyFcn=|
      | %break library link
      | link_status = get_param(gcb, 'LinkStatus');
      | if strcmp(link_status, 'resolved') || strcmp(link_status, 'inactive')
      |     set_param(gcb, 'LinkStatus', 'none');
      | end
      | 
      | cd_remote_callback('copy');
  Remote Signals : S-Function  FunctionName=cd_get_set_signals  Parameters=block_name,op_mode,port_vector,sample_time  EnableBusSupport=off  mask(CD_RemoteSignals){block_name='Test', op_mode=Write the input, port_vector=[4 4], sample_time=-1}
      mask prompts: block_name "Block Name"; op_mode "Operating Mode"; port_vector "Port dimension vector"; sample_time "Sample time"
      mask help: Allows an Embedded Matlab block to remotely set the inputs to the function-call subsystem that it calls.
      settings: CopyFcn=UAVdesign_net_cd_get_set_signals_callback(gcb);
      mask StyleString: edit,popup(Write the input|Read the output|Generate the signals ID),edit,edit
      mask Display: disp(block_name)

== system UAVdesign_net/Utilities/Kalman Filter ==
  Discrete-Continuous EKF : S-Function  FunctionName=kalman_filter_sfun  Parameters=sample_time  EnableBusSupport=off  mask(KalmanFilter){sample_time=1}
      mask prompts: sample_time "Discrete Sample Time"
      mask help:
      | Discrete-Continuous Kalman filter.
      | The x vector and P matrix have to be concatenated into a single vector before they are fed to the Kalman Filter block.
      | The outputs of the Kalman Filter block have to be transformed back into the x vector and P matrix before being used somewhere else in the model.
      mask Display:
      | port_label('input', 1, 'x_0', 'texmode', 'on')
      | port_label('input', 2, 'x_k^+', 'texmode', 'on')
      | port_label('input', 3, 'x^\bullet', 'texmode', 'on')
      | 
      | port_label('output', 1, 'exec', 'texmode', 'on')
      | port_label('output', 2, 'x_k^-', 'texmode', 'on')
      | port_label('output', 3, 'x', 'texmode', 'on')
  Discrete-Continuous Trigger : S-Function  FunctionName=trigger_mix_sr_sfun  Parameters=sample_time  EnableBusSupport=off  mask(DiscreteContinuousTrigger){sample_time=-1}
      mask prompts: sample_time "Input Sample Time"
      mask help:
      | This block generates a pulse at the beginning of a continuous-time integration step.
      | This happens only when the discrete-time input is one and only at the discrete time step.
      | The output becomes zero the rest of the major time step at the output side.
      mask Display:
      | port_label('input', 1, 'Enable');
      | port_label('Output', 1, 'Trigger');

== system UAVdesign_net/Utilities/Math ==
  3x3 Cross Product : Subsystem
      mask Type: CrossProduct
      mask Description: Calculate the cross product of two 3-by-1 vectors.
      mask Display:
      | text(.5,.5,'Cross\nProduct\nC = AxB', ...
      | 	'HorizontalAlignment','Center',...
      | 	'VerticalAlignment','middle')
  Adjoint of 3x3 Matrix : Subsystem
      mask Type: Adjoint of 3x3 matrix
      mask Description: Compute the adjoint matrix for the input matrix.
      mask Help: web(asbhelp);
      mask Display:
      | text(.5,.5,'adj(A)\n(3x3)',...
      | 	'horizontalalignment','center');
  Create 3x3 Matrix : Subsystem
      mask Type: Create 3x3 Matrix
      mask Description:
      | Create a 3-by-3 matrix from nine input values. Each input corresponds to an element of the matrix.
      | 
      | For example, the input labeled A21 is the entry in the second row and first column of the matrix.
      mask Display:
      | port_label('input',1,'A_{11}','texmode','on');
      | port_label('input',2,'A_{12}','texmode','on');
      | port_label('input',3,'A_{13}','texmode','on');
      | port_label('input',4,'A_{21}','texmode','on');
      | port_label('input',5,'A_{22}','texmode','on');
      | port_label('input',6,'A_{23}','texmode','on');
      | port_label('input',7,'A_{31}','texmode','on');
      | port_label('input',8,'A_{32}','texmode','on');
      | port_label('input',9,'A_{33}','texmode','on');
      | port_label('output',1,'A','texmode','on');
  Determinant of 3x3 Matrix : Subsystem
      mask Type: Determinant of 3x3 Matrix
      mask Description: Compute the determinant of 3x3 matrix.
      mask Display:
      | text(.5,.5,'det(A)\n(3x3)',...
      | 	'horizontalalignment','center');
  Invert  3x3 Matrix : Subsystem
      mask Type: Invert 3x3 Matrix
      mask Description: Compute the inverse of 3-by-3 matrix using determinant formula.
      mask Display:
      | text(.5,.5,'inv(A)\n(3x3)',...
      | 	'horizontalalignment','center');
  Quaternion Conjugate : Subsystem
      mask Type: Quaternion Conjugate
      mask Description: Calculate the conjugate of a quaternion.
  Quaternion Derivative : Subsystem  mask(Quaternion Derivative){k_quat=1}
      mask prompts: k_quat "Normalization gain"
      mask help: Calculates the derivative of a quaternion.
      mask Display:
      | port_label('input', 1, '\omega_b (xyz)','texmode','on');
      | port_label('input', 2, 'q','texmode','on');
      | port_label('output', 1, 'q^\bullet','texmode','on');
  Quaternion Division : Subsystem
      mask Type: Quaternion Division
      mask Description: Divide a quaternion by another quaternion.
  Quaternion Integrator : S-Function  FunctionName=quaternionintegrator  Parameters=x0external, x0, dirchange  EnableBusSupport=off  mask(QuaternionIntegrator){x0external=off, x0=[1 0 0 0], dirchange=off}
      mask prompts: x0external "Initial conditions supplied externally"; x0 "Initial conditions"; dirchange "Rotation direction changes during integration"
      mask help: Integrates rotation quaternions. Keeps the norm equal to one.
      mask init:
      | if x0external,
      |     if dirchange,
      |         set_param(gcb, 'MaskDisplay', 'disp(''\fontsize{16}\int'', ''texmode'', ''on''); port_label(''input'', 2, ''\omega^{\bullet}'', ''texmode'', ''on'');port_label(''input'', 3, ''x_0'', ''texmode'', ''on'')');
      |     else
      |         set_param(gcb, 'MaskDisplay', 'disp(''\fontsize{16}\int'', ''texmode'', ''on''); port_label(''input'', 2, ''x_0'', ''texmode'', ''on'')');
      |     end
      | else
      |     if dirchange,
      |         set_param(gcb, 'MaskDisplay', 'disp(''\fontsize{16}\int'', ''texmode'', ''on''); port_label(''input'', 2, ''\omega^{\bullet}'', ''texmode'', ''on'')');
      |     else
      |         set_param(gcb, 'MaskDisplay', 'disp(''\fontsize{16}\int'', ''texmode'', ''on'')');
      |     end
      | end
      | 
      | maskval = get_param(gcb, 'MaskValues');
      | visibility = get_param(gcb, 'MaskVisibilities');
      | if strcmp(maskval{1}, 'on'),
      |     visibility{2} = 'off';
      | else
      | 	visibility{2} = 'on';
      | end
      | set_param(gcb, 'MaskVisibilities', visibility);
      mask CallbackString:
      | maskval = get_param(gcb, 'MaskValues');
      | visibility = get_param(gcb, 'MaskVisibilities');
      | if strcmp(maskval{1}, 'on'),
      |     visibility{2} = 'off';
      | else
      | 	visibility{2} = 'on';
      | end
      | set_param(gcb, 'MaskVisibilities', visibility);||
      mask Display: disp('\fontsize{16}\int', 'texmode', 'on')
  Quaternion Inverse : Subsystem
      mask Type: Quaternion Inverse
      mask Description: Calculate inverse of a quaternion.
  Quaternion Minimum Rotation : Subsystem
      mask Type: Quaternion Minimum Rotation
      mask Description: Output q or -q such that the rotation angle is less than pi.
  Quaternion Modulus : Subsystem
      mask Type: Quaternion Modulus
      mask Description: Calculate the modulus of a quaternion.
  Quaternion Multiplication : Subsystem
      mask Type: Quaternion Multiplication
      mask Description: Calculate the product of two quaternions.
      mask Display:
      | port_label('input', 1, 'q');
      | port_label('input', 2, 'r');
      | port_label('output', 1, 'q\timesr','texmode','on');
  Quaternion Norm : Subsystem
      mask Type: Quaternion Norm
      mask Description: Calculate the norm of a quaternion.
  Quaternion Normalize : Subsystem
      mask Type: Quaternion Normalize
      mask Description: Normalize a quaternion.
  Quaternion Rotation (B<E) : Subsystem
      mask Type: Quaternion Rotation
      mask Description: Rotate a vector by a quaternion.
      mask Display:
      | port_label('input', 1, 'q');
      | port_label('input', 2, 'v');
      | port_label('output', 1, 'q^*\timesv\timesq','texmode','on');
  Quaternion Rotation (E<B) : Subsystem
      mask Type: Quaternion Rotation
      mask Description: Rotate a vector by a quaternion.
      mask Display:
      | port_label('input', 1, 'q');
      | port_label('input', 2, 'v');
      | port_label('output', 1, 'q\timesv\timesq^*','texmode','on');
  Quaternion to Vector : Subsystem
      mask Type: Quaternion to Vector
      mask Description: Converts a quaternion to a 3-component vector.
  SinCos : Subsystem
      mask Type: SinCos
      mask Description: Compute the sine and cosine of input, u. u is in radians.
      mask Display:
      | port_label('output',1,'sin(u)','texmode','on');
      | port_label('output',2,'cos(u)','texmode','on');
  Transpose : Subsystem
      mask Type: MathTranspose
      mask Description: Transpose of a matrix
      mask Display: disp('A^T', 'texmode', 'on')
  Vector to Quaternion : Subsystem
      mask Type: Vector to Quaternion
      mask Description: Converts a 3-component vector to a quaternion.

== system UAVdesign_net/Utilities/Numeric Perturbation ==
  Find Jacobian : S-Function  FunctionName=jacobian_sfun  Parameters=NumFInputs, NumFOutputs, RunOnce, SampleTime  SFunctionModules='matrixlib'  EnableBusSupport=off  mask(Trim){NumFInputs=4, NumFOutputs=4, RunOnce=on, SampleTime=-1}
      mask prompts: NumFInputs "Number of inputs to the function (dim x)"; NumFOutputs "Number of outputs of the function (dim y)"; RunOnce "Run Once"; SampleTime "Sample Time"
      mask help:
      | Searches for c such that
      | a = f(c)
      | equals zero (a=0).
      mask Display:
      | port_label('input', 1, 'x 0', 'texmode', 'on')
      | port_label('input', 2, 'y in', 'texmode', 'on')
      | port_label('output', 1, 'fun', 'texmode', 'on')
      | port_label('output', 2, 'J', 'texmode', 'on')
      | port_label('output', 3, 'x out', 'texmode', 'on')
  Find Trim : S-Function  FunctionName=trim_sfun  Parameters=NumFInputs, NumFOutputs, RunOnce, SampleTime  SFunctionModules='matrixlib'  EnableBusSupport=off  mask(Trim){NumFInputs=4, NumFOutputs=4, RunOnce=on, SampleTime=-1}
      mask prompts: NumFInputs "Dimension of c"; NumFOutputs "Dimension of a"; RunOnce "Run Once"; SampleTime "Sample Time"
      mask help:
      | Searches for c such that
      | a = f(c)
      | equals zero (a=0).
      mask Display:
      | port_label('input', 1, 'c 0', 'texmode', 'on')
      | port_label('input', 2, 'a in', 'texmode', 'on')
      | port_label('output', 1, 'fun', 'texmode', 'on')
      | port_label('output', 2, 'c final', 'texmode', 'on')
      | port_label('output', 3, 'c out', 'texmode', 'on')

== system UAVdesign_net/Utilities/Unit Conversion ==
  Angle Conversion : Subsystem  mask(Angle Conversion){IU=deg, OU=rad}
      mask prompts: IU "Initial units:"; OU "Final units:"
      mask help: Convert units of input signal to desired output units.
      mask init:
      | slopes    = [pi/180.0 1.0 2*pi];
      | units     = {'deg', 'rad', 'rev'};
      | imode = find(strcmpi(get_param(gcbh,'IU'),units),1);
      | omode = find(strcmpi(get_param(gcbh,'OU'),units),1);
      | in_txt    = units{imode};
      | out_txt   = units{omode};
      | slope_in  = slopes(imode);
      | slope_out = slopes(omode);
      | slope     = slope_in/slope_out;
      mask StyleString: popup(deg|rad|rev),popup(deg|rad|rev)
      mask Display:
      | port_label('input',1,in_txt);
      | port_label('output',1,out_txt);
